simulink model "cascade_control"  (Simulink 3.00)
libraries: mathlib x7, execlib x5, analoglib x4, paramlib x3, reglib x3, logiclib x2, arclib x1

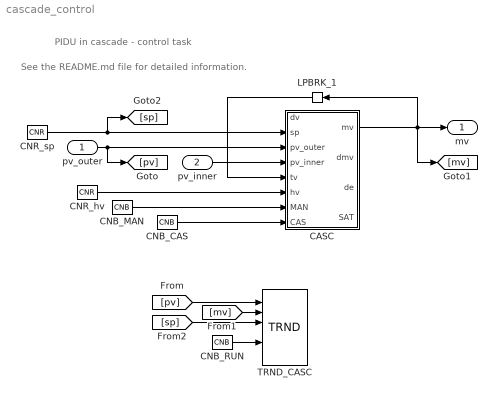
== system cascade_control ==
  note: See the README.md file for detailed information.
  note: PIDU in cascade - control task
  pv_outer : Inport  Port=1
  pv_inner : Inport  Port=2
  CASC : Subsystem
      mask Type: REX sequence
  CNB_CAS : mathlib/CNB  YCN=on
  CNB_MAN : mathlib/CNB  YCN=off
  CNB_RUN : mathlib/CNB  YCN=on
  CNR_hv : mathlib/CNR  ycn=1
  CNR_sp : mathlib/CNR  ycn=5
  LPBRK_1 : execlib/LPBRK  Orientation=left
  TRND_CASC : arclib/TRND  n=3  l=1000  btype=8  ptype1=1: Store  ptype2=1: Store  ptype3=1: Store  ptype4=1: Store  pfac=1  afac=0  arc=0  id=1  Title=Trend Title  timesrc=1
  mv : Outport  Port=1
  wires:
  CASC/1(mv) -> [mv], LPBRK_1/1, mv/1
  CNB_CAS/1 -> CASC/8(CAS)
  CNB_MAN/1 -> CASC/7(MAN)
  CNB_RUN/1 -> TRND_CASC/5
  CNR_hv/1 -> CASC/6(hv)
  CNR_sp/1 -> CASC/2(sp), [sp]
  [pv] -> TRND_CASC/1
  [mv] -> TRND_CASC/2
  [sp] -> TRND_CASC/3
  LPBRK_1/1 -> CASC/5(tv)
  pv_inner/1 -> CASC/4(pv_inner)
  pv_outer/1 -> CASC/3(pv_outer), [pv]

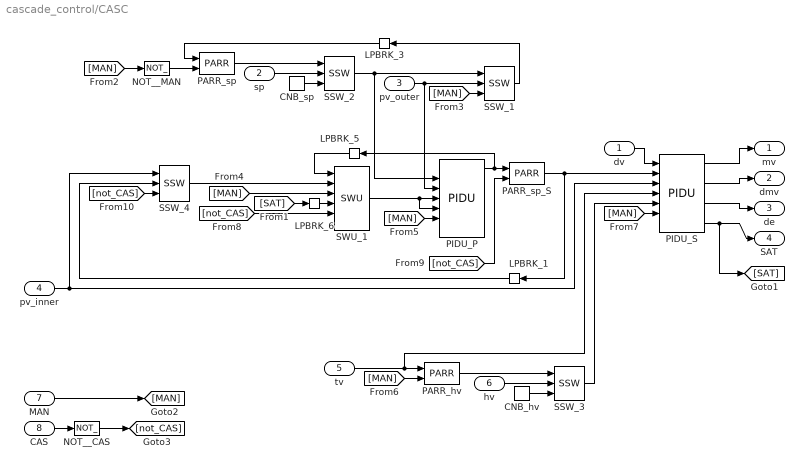
== system cascade_control/CASC ==
  dv : Inport  Port=1
  sp : Inport  Port=2
  pv_outer : Inport  Port=3
  pv_inner : Inport  Port=4
  tv : Inport  Port=5
  hv : Inport  Port=6
  MAN : Inport  Port=7
  CAS : Inport  Port=8
  CNB_hv : mathlib/CNB  YCN=off
  CNB_sp : mathlib/CNB  YCN=on
  LPBRK_1 : execlib/LPBRK  Orientation=left
  LPBRK_3 : execlib/LPBRK  Orientation=left
  LPBRK_5 : execlib/LPBRK  Orientation=left
  LPBRK_6 : execlib/LPBRK
  NOT__CAS : logiclib/NOT_
  NOT__MAN : logiclib/NOT_
  PARR_hv : paramlib/PARR  par=1  SATF=off  hilim=1  lolim=-1
  PARR_sp : paramlib/PARR  par=1  SATF=off  hilim=1  lolim=-1
  PARR_sp_S : paramlib/PARR  par=1  SATF=off  hilim=1  lolim=-1
  PIDU_P : reglib/PIDU  irtype=7: PID  RACT=off  k=0.71  ti=6  td=1.5  nd=4  b=1  c=0  tt=1  hilim=100  lolim=0  dz=0  icotype=1: Analog
  PIDU_S : reglib/PIDU  irtype=7: PID  RACT=off  k=0.04  ti=4  td=1  nd=4  b=1  c=0  tt=1  hilim=1  lolim=0  dz=0  icotype=1: Analog
  SSW_{1..4} (4 alike) : analoglib/SSW
  SWU_1 : reglib/SWU
  mv : Outport  Port=1
  dmv : Outport  Port=2
  de : Outport  Port=3
  SAT : Outport  Port=4
  wires:
  CAS/1 -> NOT__CAS/1
  CNB_hv/1 -> SSW_3/3
  CNB_sp/1 -> SSW_2/3
  [SAT] -> LPBRK_6/1
  [not_CAS] -> SSW_4/3
  [MAN] -> NOT__MAN/1
  [MAN] -> SSW_1/3
  [MAN] -> SWU_1/3
  [MAN] -> PIDU_P/6
  [MAN] -> PARR_hv/2
  [MAN] -> PIDU_S/6
  [not_CAS] -> SWU_1/5
  [not_CAS] -> PARR_sp_S/2
  LPBRK_1/1 -> SSW_4/2
  LPBRK_3/1 -> PARR_sp/1
  LPBRK_5/1 -> SWU_1/1
  LPBRK_6/1 -> SWU_1/4
  MAN/1 -> [MAN]
  NOT__CAS/1 -> [not_CAS]
  NOT__MAN/1 -> PARR_sp/2
  PARR_hv/1 -> SSW_3/1
  PARR_sp/1 -> SSW_2/1
  PARR_sp_S/1 -> LPBRK_1/1, PIDU_S/2
  PIDU_P/1 -> LPBRK_5/1, PARR_sp_S/1
  PIDU_S/1 -> mv/1
  PIDU_S/2 -> dmv/1
  PIDU_S/3 -> de/1
  PIDU_S/4 -> [SAT], SAT/1
  SSW_1/1 -> LPBRK_3/1
  SSW_2/1 -> PIDU_P/2, SSW_1/1
  SSW_3/1 -> PIDU_S/5
  SSW_4/1 -> SWU_1/2
  SWU_1/1 -> PIDU_P/4, PIDU_P/5
  dv/1 -> PIDU_S/1
  hv/1 -> SSW_3/2
  pv_inner/1 -> PIDU_S/3, SSW_4/1
  pv_outer/1 -> PIDU_P/3, SSW_1/2
  sp/1 -> SSW_2/2
  tv/1 -> PARR_hv/1, PIDU_S/4
